simulink model "NonlinearSolenoid"  (R2018a)
settings: Solver=VariableStepAuto  StartTime=0.0  StopTime=20  RelTol=1e-3
values from neighbouring files (symbols this model uses):
  alpha = 0.003725    [Linearization&MDPP.m]
  beta = 0.0005685    [Linearization&MDPP.m]
  c = 1.5    [Linearization&MDPP.m]
  rd = cell2mat(rdd)    [Linearization&MDPP.m]
  sd = cell2mat(sdd)    [Linearization&MDPP.m]
  td = cell2mat(tdd)    [Linearization&MDPP.m]
  Ts = 0.005*2*pi/fb    [Linearization&MDPP.m]
libraries: fl_lib x14, nesl_utility x5, pe_lib x1, powerlib_meascontrol x1
settings Model: Creator=Hirsa  LastModifiedBy=Hirsa

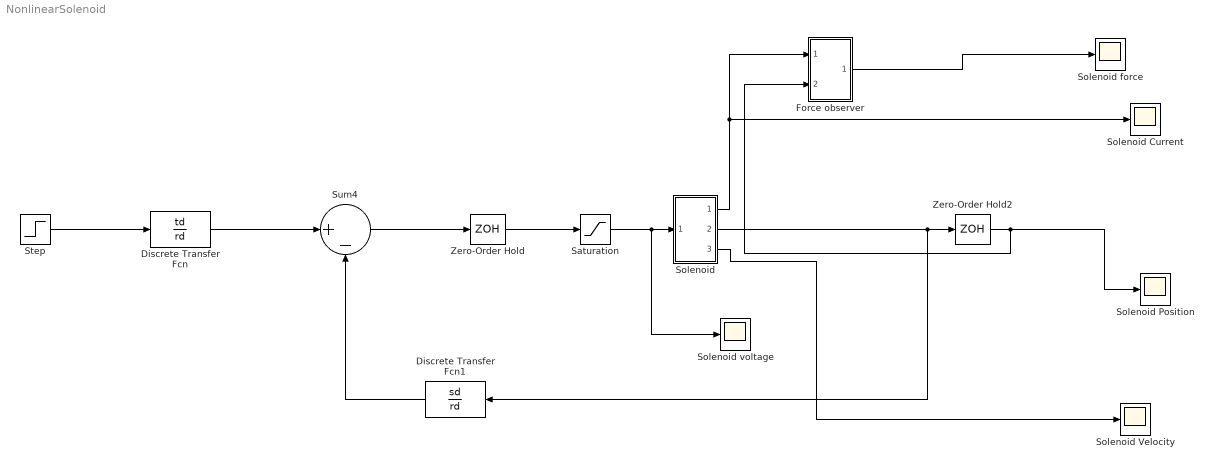
== system NonlinearSolenoid ==
  Discrete Transfer Fcn : DiscreteTransferFcn  Numerator=td  Denominator=rd  SampleTime=Ts
  Discrete Transfer Fcn1 : DiscreteTransferFcn  Numerator=sd  Denominator=rd  SampleTime=Ts
  Force observer : Subsystem
  Saturation : Saturate  UpperLimit=5  LowerLimit=-5
  Solenoid : Subsystem
  Solenoid Current : Scope
  Solenoid Position : Scope
  Solenoid Velocity : Scope
  Solenoid force : Scope
  Solenoid voltage : Scope
  Step : Step  After=0.005  SampleTime=Ts
  Sum4 : Sum  Inputs=|+-
  Zero-Order Hold : ZeroOrderHold  SampleTime=Ts
  Zero-Order Hold2 : ZeroOrderHold  SampleTime=Ts
  wires:
  Sum4/1 -> Zero-Order Hold/1
  Step/1 -> Discrete Transfer Fcn/1
  Solenoid/2(Out2) -> Discrete Transfer Fcn1/1, Zero-Order Hold2/1
  Zero-Order Hold2/1 -> Force observer/2(In2), Solenoid Position/1
  Solenoid/3(Out3) -> Solenoid Velocity/1
  Zero-Order Hold/1 -> Saturation/1
  Solenoid/1(Out1) -> Force observer/1(In1), Solenoid Current/1
  Saturation/1 -> Solenoid voltage/1, Solenoid/1(In1)
  Discrete Transfer Fcn/1 -> Sum4/1
  Discrete Transfer Fcn1/1 -> Sum4/2
  Force observer/1(Out1) -> Solenoid force/1

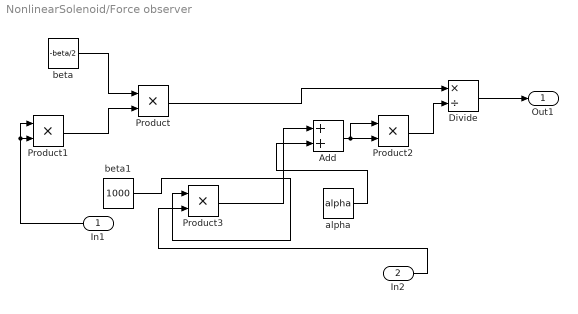
== system NonlinearSolenoid/Force observer ==
  In1 : Inport
  In2 : Inport  Port=2
  Add : Sum
  Divide : Product  Inputs=*/
  Product{,1..3} (4 alike) : Product
  alpha : Constant  Value=alpha
  beta : Constant  Value=-beta/2
  beta1 : Constant  Value=1000
  Out1 : Outport
  wires:
  Divide/1 -> Out1/1
  Product2/1 -> Divide/2
  beta/1 -> Product/1
  In1/1 -> Product1/2, Product1/1
  Add/1 -> Product2/1, Product2/2
  Product1/1 -> Product/2
  alpha/1 -> Add/2
  Product/1 -> Divide/1
  Product3/1 -> Add/1
  In2/1 -> Product3/2
  beta1/1 -> Product3/1

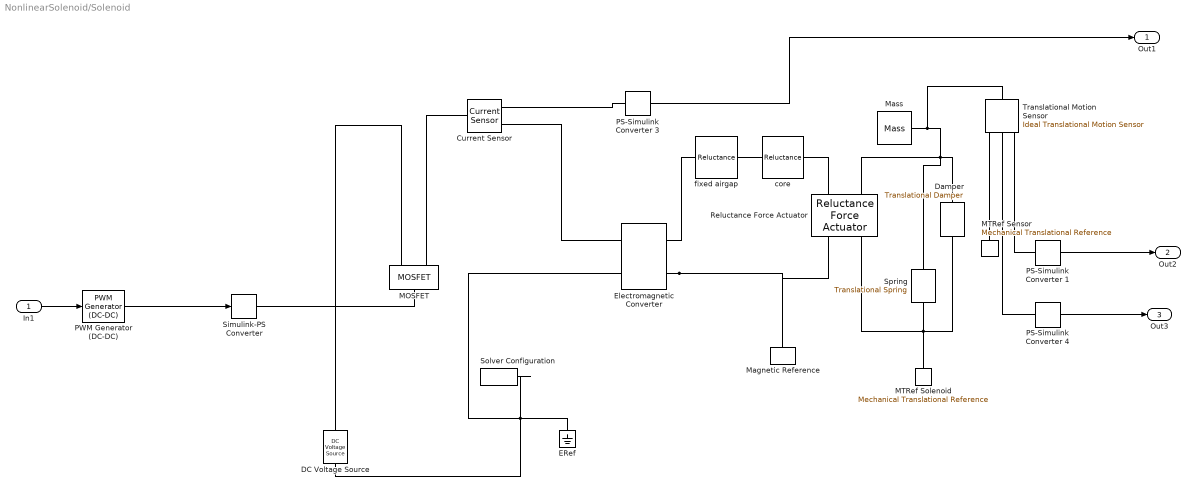
== system NonlinearSolenoid/Solenoid ==
  In1 : Inport
  Current Sensor : fl_lib/Electrical/Electrical Sensors/Current Sensor
  DC Voltage Source : fl_lib/Electrical/Electrical Sources/DC Voltage Source  v0=24 V
  Damper : fl_lib/Mechanical/Translational Elements/Translational Damper  D=c N/(m/s)  v_specify=off  v_priority=High  v=0 m/s  v_nominal_specify=off  v_nominal_unit=m/s  v_nominal_value=1  f_specify=off  f_priority=High  f=0 N  f_nominal_specify=off  f_nominal_unit=N  f_nominal_value=1
  ERef : fl_lib/Electrical/Electrical Elements/Electrical Reference
  Electromagnetic Converter : fl_lib/Magnetic/Magnetic Elements/Electromagnetic Converter  Nw=600  i_specify=off  i_priority=None  i=0 A  i_nominal_specify=off  i_nominal_unit=A  i_nominal_value=1  v_specify=off  v_priority=None  v=0 V  v_nominal_specify=off  v_nominal_unit=V  v_nominal_value=1  mmf_specify=off  mmf_priority=None  mmf=0 A  mmf_nominal_specify=off  mmf_nominal_unit=A  mmf_nominal_value=1  phi_specify=off  phi_priority=High  phi=0 Wb  phi_nominal_specify=off  phi_nominal_unit=Wb  phi_nominal_value=1
      settings: SourceProductName=Simscape  SourceProductBaseCode=SS
  MOSFET : pe_lib/Semiconductors/Fundamental Components/MOSFET  Rds=1e-6 Ohm  Goff=1e-6 1/Ohm  Vth=0 V  diode_param=2  diode_Vf=0.8 V  diode_Ron=0.001 Ohm  diode_Goff=1e-5 1/Ohm  diode_C=5e-8 F  diode_iRM=-235 A  diode_iF=300 A  diode_idot=-50 A/us  diode_trr_param=1  diode_trr_factor=3  diode_trr=15 us  diode_Qrr=1.5e+3 s*uA  thermal_loss_option=2  Voff=300 V  Tau=1e-4 s  Tj=[ 298.15 398.15 ] K  Iout_scalar=600 A  Eon_scalar=0.02286 J  Eoff_scalar=0.01714 J  Von_scalar=2.7 V  Iout_data=[ 0 10 50 100 200 400 600 ] A  Eon_data=[ 0 2.9e-4 0.00143 0.00286 0.00571 0.01314 0.02286; 0 5.7e-4 0.00263 0.00514 0.01029 0.02057 0.03029 ] J  Eoff_data=[ 0 2.1e-4 0.00107 0.00214 0.00429 0.009859999999999999 0.01714; 0 4.3e-4 0.00197 0.00386 0.00771 0.01543 0.02271 ] J  Von_data=[ 0 1.1 1.3 1.45 1.75 2.25 2.7; 0 1 1.15 1.35 1.7 2.35 3 ] V
      settings: SourceProductName=Simscape Power Systems  SourceProductBaseCode=PS
  MTRef Sensor : fl_lib/Mechanical/Translational Elements/Mechanical Translational Reference
  MTRef Solenoid : fl_lib/Mechanical/Translational Elements/Mechanical Translational Reference
  Magnetic Reference : fl_lib/Magnetic/Magnetic Elements/Magnetic Reference
      settings: SourceProductName=Simscape  SourceProductBaseCode=SS
  Mass : fl_lib/Mechanical/Translational Elements/Mass  mass=m kg  v_specify=off  v_priority=High  v=0 m/s  v_nominal_specify=off  v_nominal_unit=m/s  v_nominal_value=1  f_specify=off  f_priority=High  f=0 N  f_nominal_specify=off  f_nominal_unit=N  f_nominal_value=1
  PS-Simulink Converter 1 : nesl_utility/PS-Simulink Converter  PhysicalDomain=network_engine_domain  SubClassName=ps_output  LeftPortType=input  RightPortType=output  PseudoPeriodic=off  Frequencies=[]  Unit=m  AffineConversion=off
  PS-Simulink Converter 3 : nesl_utility/PS-Simulink Converter  PhysicalDomain=network_engine_domain  SubClassName=ps_output  LeftPortType=input  RightPortType=output  PseudoPeriodic=off  Frequencies=[]  Unit=A  AffineConversion=off
  PS-Simulink Converter 4 : nesl_utility/PS-Simulink Converter  PhysicalDomain=network_engine_domain  SubClassName=ps_output  LeftPortType=input  RightPortType=output  PseudoPeriodic=off  Frequencies=[]  Unit=m/s  AffineConversion=off
  PWM Generator (DC-DC) : powerlib_meascontrol/Pulse & Signal Generators/PWM Generator (DC-DC)  Fsw=10000  Ts=Ts
  Reluctance Force Actuator : fl_lib/Magnetic/Magnetic Elements/Reluctance Force Actuator  x0=11 mm  xmin=1 mm  CSA=pi*(20^2) mm^2  mur=1000  K_contact=1e8 N/m  D_contact=150000 N/(m/s)  mmf_specify=off  mmf_priority=None  mmf=0 A  mmf_nominal_specify=off  mmf_nominal_unit=A  mmf_nominal_value=1  phi_specify=off  phi_priority=None  phi=0 Wb  phi_nominal_specify=off  phi_nominal_unit=Wb  phi_nominal_value=1  f_specify=off  f_priority=None  f=0 N  f_nominal_specify=off  f_nominal_unit=N  f_nominal_value=1  u_specify=off  u_priority=None  u=0 m/s  u_nominal_specify=off  u_nominal_unit=m/s  u_nominal_value=1
      settings: SourceProductName=Simscape  SourceProductBaseCode=SS
  Simulink-PS Converter : nesl_utility/Simulink-PS Converter  PhysicalDomain=network_engine_domain  SubClassName=ps_input  LeftPortType=input  RightPortType=output  PseudoPeriodic=off  Frequencies=[]  NoiseDistribution=none  NoiseParameters=[]  Unit=V  AffineConversion=off  FilteringAndDerivatives=provide  SimscapeFilterOrder=1  InputFilterTimeConstant=0.001  UdotUserProvided=0
  Solver Configuration : nesl_utility/Solver Configuration  PhysicalDomain=network_engine_domain  SubClassName=solver  LeftPortType=input  RightPortType=generic  Tones=[]  Harmonics=[]  SimulateNoise=off  Profile=off  UseLocalSampling=off  EnableSwitchedLinearOptims=on  FrequencyDomain=off  UseCCode=off  RelTol=0.001  AbsTol=1e-06  MinStep=1e-09  ToWorkspace=off  RevertToSquareIcSolve=off  NumHomotopyIterations=100  PhasorMode=off  PhasorModeNumHarmonics=1  DoDC=off  ResidualTolerance=1e-9  UseLocalSolver=off  LocalSolverChoice=NE_BACKWARD_EULER_ADVANCER  LocalSolverSampleTime=.001  DoFixedCost=off  MaxNonlinIter=3  MaxModeIter=2  LinearAlgebra=Sparse  EquationFormulation=NE_TIME_EF  DelaysMemoryBudget=1024  AutomaticFiltering=on  FilteringTimeConstant=0.001
  Spring : fl_lib/Mechanical/Translational Elements/Translational Spring  spr_rate=k N/m  v_specify=off  v_priority=High  v=0 m/s  v_nominal_specify=off  v_nominal_unit=m/s  v_nominal_value=1  f_specify=off  f_priority=High  f=0 N  f_nominal_specify=off  f_nominal_unit=N  f_nominal_value=1  x_specify=off  x_priority=High  x=1 m  x_nominal_specify=off  x_nominal_unit=m  x_nominal_value=1
  Translational Motion Sensor : fl_lib/Mechanical/Mechanical Sensors/Ideal Translational Motion Sensor  offset=10 mm
  core : fl_lib/Magnetic/Magnetic Elements/Reluctance  g=5 mm  CSA=pi*(40^2)/4 mm^2  mur=1000  phi_specify=off  phi_priority=None  phi=0 Wb  phi_nominal_specify=off  phi_nominal_unit=Wb  phi_nominal_value=1  mmf_specify=off  mmf_priority=None  mmf=0 A  mmf_nominal_specify=off  mmf_nominal_unit=A  mmf_nominal_value=1
      settings: SourceProductName=Simscape  SourceProductBaseCode=SS
  fixed airgap : fl_lib/Magnetic/Magnetic Elements/Reluctance  g=3 mm  CSA=pi*(40)*8 mm^2  mur=1  phi_specify=off  phi_priority=None  phi=0 Wb  phi_nominal_specify=off  phi_nominal_unit=Wb  phi_nominal_value=1  mmf_specify=off  mmf_priority=None  mmf=0 A  mmf_nominal_specify=off  mmf_nominal_unit=A  mmf_nominal_value=1
      settings: SourceProductName=Simscape  SourceProductBaseCode=SS
  Out1 : Outport
  Out2 : Outport  Port=2
  Out3 : Outport  Port=3
  wires:
  PS-Simulink Converter 4/1 -> Out3/1
  PS-Simulink Converter 1/1 -> Out2/1
  In1/1 -> PWM Generator (DC-DC)/1
  PS-Simulink Converter 3/1 -> Out1/1
  PWM Generator (DC-DC)/1 -> Simulink-PS Converter/1
  connections:
  Translational Motion Sensor/LConn1 -- Mass/LConn1 -- Spring/LConn1 -- Damper/LConn1 -- Reluctance Force Actuator/LConn2
  ERef/LConn1 -- Solver Configuration/RConn1 -- Electromagnetic Converter/LConn2 -- DC Voltage Source/RConn1
  fixed airgap/LConn1 -- Electromagnetic Converter/RConn1
  Damper/RConn1 -- Spring/RConn1 -- Reluctance Force Actuator/RConn2 -- MTRef Solenoid/LConn1
  Electromagnetic Converter/RConn2 -- Magnetic Reference/LConn1 -- Reluctance Force Actuator/RConn1
  Translational Motion Sensor/RConn1 -- MTRef Sensor/LConn1
  core/RConn1 -- Reluctance Force Actuator/LConn1
  Translational Motion Sensor/RConn3 -- PS-Simulink Converter 1/LConn1
  PS-Simulink Converter 3/LConn1 -- Current Sensor/RConn1
  PS-Simulink Converter 4/LConn1 -- Translational Motion Sensor/RConn2
  fixed airgap/RConn1 -- core/LConn1
  DC Voltage Source/LConn1 -- MOSFET/RConn1
  MOSFET/RConn2 -- Current Sensor/LConn1
  Simulink-PS Converter/RConn1 -- MOSFET/LConn1
  Current Sensor/RConn2 -- Electromagnetic Converter/LConn1
